simulink model "System_Design_Quadrocopter"  (Simulink 7.5)
settings: Solver=ode45  StartTime=0.0  StopTime=30  RelTol=1e-3
values from neighbouring files (symbols this model uses):
  phi0 = 0.15    [Quadrocopter_control_Driver.m]    (also in calc_stability.m = 0)
  r_phi0 = 0    [Quadrocopter_control_Driver.m]    (also in calc_stability.m)
  r_psi0 = 0    [Quadrocopter_control_Driver.m]    (also in calc_stability.m)
  r_theta0 = 0    [Quadrocopter_control_Driver.m]    (also in calc_stability.m)
  theta0 = 0.15    [Quadrocopter_control_Driver.m]    (also in calc_stability.m = 0)
  Ts = 0.01    [Reglerauslegung.m]    (also in Test_Reglerauslegung.m)
undefined symbols (not defined in the file or in its folder): bodyCtrl_phiCtrl_KD, bodyCtrl_phiCtrl_KI, bodyCtrl_phiCtrl_KP, bodyCtrl_rphiCtrl_KD, bodyCtrl_rphiCtrl_KI, bodyCtrl_rphiCtrl_KP, bodyCtrl_rpsiCtrl_KD, bodyCtrl_rpsiCtrl_KI, bodyCtrl_rpsiCtrl_KP, bodyCtrl_rthetaCtrl_KD, bodyCtrl_rthetaCtrl_KI, bodyCtrl_rthetaCtrl_KP, bodyCtrl_thetaCtrl_KD, bodyCtrl_thetaCtrl_KI, bodyCtrl_thetaCtrl_KP, boom, f1, f2, f3, f4, f5, g, I_x, I_y, I_z, m, positionCtrl_rpsiCtrl_KD, positionCtrl_rpsiCtrl_KI, positionCtrl_rpsiCtrl_KP, sigbuilder_block, speed, thrust, Ts_Opt
libraries: simulink x39, dspobslib x4, Copter_Library x3, Control_lib x1, sdolib x1
(part 2 of 4)

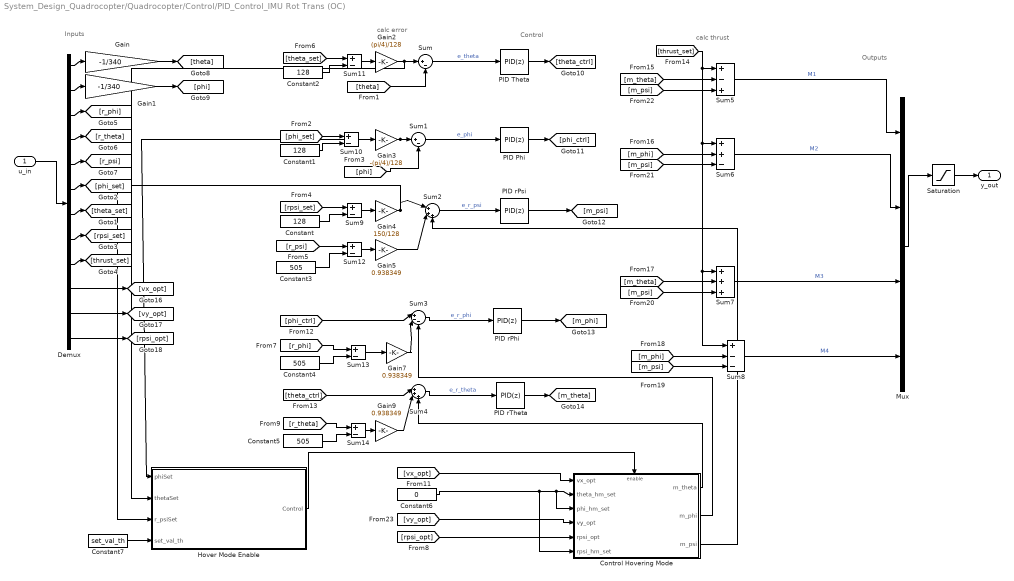
== system System_Design_Quadrocopter/Quadrocopter/Control/PID_Control_IMU Rot Trans (OC) ==
  note: calc thrust
  note: Control
  note: Outputs
  note: calc error
  note: Inputs
  u_in : Inport  OutDataType=fixdt(1, 16)  OutScaling=2^0
  Constant : Constant  Value=128  OutDataType=fixdt(1, 16)  OutScaling=2^0
  Constant1 : Constant  Value=128  OutDataType=fixdt(1, 16)  OutScaling=2^0
  Constant2 : Constant  Value=128  OutDataType=fixdt(1, 16)  OutScaling=2^0
  Constant3 : Constant  Value=505  OutDataType=fixdt(1, 16)  OutScaling=2^0
  Constant4 : Constant  Value=505  OutDataType=fixdt(1, 16)  OutScaling=2^0
  Constant5 : Constant  Value=505  OutDataType=fixdt(1, 16)  OutScaling=2^0
  Constant6 : Constant  Value=0  OutDataType=fixdt(1, 16)  OutScaling=2^0
  Constant7 : Constant  Value=set_val_th  OutDataType=fixdt(1, 16)  OutScaling=2^0
  Control Hovering Mode : Subsystem
  Demux : Demux  Outputs=12
  Gain : Gain  Gain=-1/340  ParameterDataType=fixdt(1, 16)  ParameterScaling=2^0  OutDataType=fixdt(1, 16)  OutScaling=2^0
  Gain1 : Gain  Gain=-1/340  ParameterDataType=fixdt(1, 16)  ParameterScaling=2^0  OutDataType=fixdt(1, 16)  OutScaling=2^0
  Gain2 : Gain  Gain=(pi/4)/128  ParameterDataType=fixdt(1, 16)  ParameterScaling=2^0  OutDataType=fixdt(1, 16)  OutScaling=2^0
  Gain3 : Gain  Gain=-(pi/4)/128  ParameterDataType=fixdt(1, 16)  ParameterScaling=2^0  OutDataType=fixdt(1, 16)  OutScaling=2^0
  Gain4 : Gain  Gain=150/128  ParameterDataType=fixdt(1, 16)  ParameterScaling=2^0  OutDataType=fixdt(1, 16)  OutScaling=2^0
  Gain5 : Gain  Gain=0.938349  ParameterDataType=fixdt(1, 16)  ParameterScaling=2^0  OutDataType=fixdt(1, 16)  OutScaling=2^0
  Gain7 : Gain  Gain=0.938349  ParameterDataType=fixdt(1, 16)  ParameterScaling=2^0  OutDataType=fixdt(1, 16)  OutScaling=2^0
  Gain9 : Gain  Gain=0.938349  ParameterDataType=fixdt(1, 16)  ParameterScaling=2^0  OutDataType=fixdt(1, 16)  OutScaling=2^0
  Hover Mode Enable : Stateflow chart  TreatAsAtomicUnit=on
  Mux : Mux
  PID Phi : simulink/Continuous/PID Controller  DialogController=pidpack.PIDConfig.pidDDGCreate  DialogControllerArgs=DataTag9  SystemSampleTime=-1  Controller=PID  TimeDomain=Discrete-time  SampleTime=Ts  IntegratorMethod=Forward Euler  FilterMethod=Forward Euler  Form=Ideal  P=150  I=0.5  D=0  N=0  InitialConditionSource=internal  InitialConditionForIntegrator=0  InitialConditionForFilter=0  ExternalReset=none  ZeroCross=off  LimitOutput=off  UpperSaturationLimit=inf  LowerSaturationLimit=-inf  LinearizeAsGain=off  AntiWindupMode=none  Kb=1  TrackingMode=off  Kt=1  PParamMin=[]  PParamMax=[]  IParamMin=[]  IParamMax=[]  DParamMin=[]  DParamMax=[]  NParamMin=[]  NParamMax=[]  KbParamMin=[]  KbParamMax=[]  KtParamMin=[]  KtParamMax=[]  POutMin=[]  POutMax=[]  IOutMin=[]  IOutMax=[]  DOutMin=[]  DOutMax=[]  NOutMin=[]  NOutMax=[]  KbOutMin=[]  KbOutMax=[]  KtOutMin=[]  KtOutMax=[]  IntegratorOutMin=[]  IntegratorOutMax=[]  FilterOutMin=[]  FilterOutMax=[]  SumOutMin=[]  SumOutMax=[]  SumI1OutMin=[]  SumI1OutMax=[]  SumI2OutMin=[]  SumI2OutMax=[]  SumI3OutMin=[]  SumI3OutMax=[]  SumDOutMin=[]  SumDOutMax=[]  SaturationOutMin=[]  SaturationOutMax=[]  IntegratorContinuousStateAttributes=''  IntegratorStateMustResolveToSignalObject=off  IntegratorRTWStateStorageClass=Auto  FilterContinuousStateAttributes=''  FilterStateMustResolveToSignalObject=off  FilterRTWStateStorageClass=Auto
  PID Theta : simulink/Continuous/PID Controller  DialogController=pidpack.PIDConfig.pidDDGCreate  DialogControllerArgs=DataTag10  SystemSampleTime=-1  Controller=PID  TimeDomain=Discrete-time  SampleTime=Ts  IntegratorMethod=Forward Euler  FilterMethod=Forward Euler  Form=Ideal  P=150  I=0.5  D=0  N=0  InitialConditionSource=internal  InitialConditionForIntegrator=0  InitialConditionForFilter=0  ExternalReset=none  ZeroCross=off  LimitOutput=off  UpperSaturationLimit=inf  LowerSaturationLimit=-inf  LinearizeAsGain=off  AntiWindupMode=none  Kb=1  TrackingMode=off  Kt=1  PParamMin=[]  PParamMax=[]  IParamMin=[]  IParamMax=[]  DParamMin=[]  DParamMax=[]  NParamMin=[]  NParamMax=[]  KbParamMin=[]  KbParamMax=[]  KtParamMin=[]  KtParamMax=[]  POutMin=[]  POutMax=[]  IOutMin=[]  IOutMax=[]  DOutMin=[]  DOutMax=[]  NOutMin=[]  NOutMax=[]  KbOutMin=[]  KbOutMax=[]  KtOutMin=[]  KtOutMax=[]  IntegratorOutMin=[]  IntegratorOutMax=[]  FilterOutMin=[]  FilterOutMax=[]  SumOutMin=[]  SumOutMax=[]  SumI1OutMin=[]  SumI1OutMax=[]  SumI2OutMin=[]  SumI2OutMax=[]  SumI3OutMin=[]  SumI3OutMax=[]  SumDOutMin=[]  SumDOutMax=[]  SaturationOutMin=[]  SaturationOutMax=[]  IntegratorContinuousStateAttributes=''  IntegratorStateMustResolveToSignalObject=off  IntegratorRTWStateStorageClass=Auto  FilterContinuousStateAttributes=''  FilterStateMustResolveToSignalObject=off  FilterRTWStateStorageClass=Auto
  PID rPhi : simulink/Continuous/PID Controller  DialogController=pidpack.PIDConfig.pidDDGCreate  DialogControllerArgs=DataTag11  SystemSampleTime=-1  Controller=PID  TimeDomain=Discrete-time  SampleTime=Ts  IntegratorMethod=Forward Euler  FilterMethod=Forward Euler  Form=Ideal  P=60  I=0.5  D=0  N=0  InitialConditionSource=internal  InitialConditionForIntegrator=0  InitialConditionForFilter=0  ExternalReset=none  ZeroCross=off  LimitOutput=off  UpperSaturationLimit=inf  LowerSaturationLimit=-inf  LinearizeAsGain=off  AntiWindupMode=none  Kb=1  TrackingMode=off  Kt=1  PParamMin=[]  PParamMax=[]  IParamMin=[]  IParamMax=[]  DParamMin=[]  DParamMax=[]  NParamMin=[]  NParamMax=[]  KbParamMin=[]  KbParamMax=[]  KtParamMin=[]  KtParamMax=[]  POutMin=[]  POutMax=[]  IOutMin=[]  IOutMax=[]  DOutMin=[]  DOutMax=[]  NOutMin=[]  NOutMax=[]  KbOutMin=[]  KbOutMax=[]  KtOutMin=[]  KtOutMax=[]  IntegratorOutMin=[]  IntegratorOutMax=[]  FilterOutMin=[]  FilterOutMax=[]  SumOutMin=[]  SumOutMax=[]  SumI1OutMin=[]  SumI1OutMax=[]  SumI2OutMin=[]  SumI2OutMax=[]  SumI3OutMin=[]  SumI3OutMax=[]  SumDOutMin=[]  SumDOutMax=[]  SaturationOutMin=[]  SaturationOutMax=[]  IntegratorContinuousStateAttributes=''  IntegratorStateMustResolveToSignalObject=off  IntegratorRTWStateStorageClass=Auto  FilterContinuousStateAttributes=''  FilterStateMustResolveToSignalObject=off  FilterRTWStateStorageClass=Auto
  PID rPsi : simulink/Continuous/PID Controller  DialogController=pidpack.PIDConfig.pidDDGCreate  DialogControllerArgs=DataTag12  SystemSampleTime=-1  Controller=PID  TimeDomain=Discrete-time  SampleTime=Ts  IntegratorMethod=Forward Euler  FilterMethod=Forward Euler  Form=Ideal  P=60  I=0  D=0  N=0  InitialConditionSource=internal  InitialConditionForIntegrator=0  InitialConditionForFilter=0  ExternalReset=none  ZeroCross=off  LimitOutput=off  UpperSaturationLimit=inf  LowerSaturationLimit=-inf  LinearizeAsGain=off  AntiWindupMode=none  Kb=1  TrackingMode=off  Kt=1  PParamMin=[]  PParamMax=[]  IParamMin=[]  IParamMax=[]  DParamMin=[]  DParamMax=[]  NParamMin=[]  NParamMax=[]  KbParamMin=[]  KbParamMax=[]  KtParamMin=[]  KtParamMax=[]  POutMin=[]  POutMax=[]  IOutMin=[]  IOutMax=[]  DOutMin=[]  DOutMax=[]  NOutMin=[]  NOutMax=[]  KbOutMin=[]  KbOutMax=[]  KtOutMin=[]  KtOutMax=[]  IntegratorOutMin=[]  IntegratorOutMax=[]  FilterOutMin=[]  FilterOutMax=[]  SumOutMin=[]  SumOutMax=[]  SumI1OutMin=[]  SumI1OutMax=[]  SumI2OutMin=[]  SumI2OutMax=[]  SumI3OutMin=[]  SumI3OutMax=[]  SumDOutMin=[]  SumDOutMax=[]  SaturationOutMin=[]  SaturationOutMax=[]  IntegratorContinuousStateAttributes=''  IntegratorStateMustResolveToSignalObject=off  IntegratorRTWStateStorageClass=Auto  FilterContinuousStateAttributes=''  FilterStateMustResolveToSignalObject=off  FilterRTWStateStorageClass=Auto
  PID rTheta : simulink/Continuous/PID Controller  DialogController=pidpack.PIDConfig.pidDDGCreate  DialogControllerArgs=DataTag13  SystemSampleTime=-1  Controller=PID  TimeDomain=Discrete-time  SampleTime=Ts  IntegratorMethod=Forward Euler  FilterMethod=Forward Euler  Form=Ideal  P=60  I=0.5  D=0  N=0  InitialConditionSource=internal  InitialConditionForIntegrator=0  InitialConditionForFilter=0  ExternalReset=none  ZeroCross=off  LimitOutput=off  UpperSaturationLimit=inf  LowerSaturationLimit=-inf  LinearizeAsGain=off  AntiWindupMode=none  Kb=1  TrackingMode=off  Kt=1  PParamMin=[]  PParamMax=[]  IParamMin=[]  IParamMax=[]  DParamMin=[]  DParamMax=[]  NParamMin=[]  NParamMax=[]  KbParamMin=[]  KbParamMax=[]  KtParamMin=[]  KtParamMax=[]  POutMin=[]  POutMax=[]  IOutMin=[]  IOutMax=[]  DOutMin=[]  DOutMax=[]  NOutMin=[]  NOutMax=[]  KbOutMin=[]  KbOutMax=[]  KtOutMin=[]  KtOutMax=[]  IntegratorOutMin=[]  IntegratorOutMax=[]  FilterOutMin=[]  FilterOutMax=[]  SumOutMin=[]  SumOutMax=[]  SumI1OutMin=[]  SumI1OutMax=[]  SumI2OutMin=[]  SumI2OutMax=[]  SumI3OutMin=[]  SumI3OutMax=[]  SumDOutMin=[]  SumDOutMax=[]  SaturationOutMin=[]  SaturationOutMax=[]  IntegratorContinuousStateAttributes=''  IntegratorStateMustResolveToSignalObject=off  IntegratorRTWStateStorageClass=Auto  FilterContinuousStateAttributes=''  FilterStateMustResolveToSignalObject=off  FilterRTWStateStorageClass=Auto
  Saturation : Saturate  UpperLimit=255  LowerLimit=0  OutDataType=fixdt(1, 16)  OutScaling=2^0
  Sum : Sum  Inputs=|+-  OutDataType=fixdt(1, 16)  OutScaling=2^0
  Sum1 : Sum  Inputs=|+-  OutDataType=fixdt(1, 16)  OutScaling=2^0
  Sum{9..14} (6 alike) : Sum  Inputs=+-  OutDataType=fixdt(1, 16)  OutScaling=2^0
  Sum2 : Sum  Inputs=|+++  OutDataType=fixdt(1, 16)  OutScaling=2^0
  Sum3 : Sum  Inputs=|+--  OutDataType=fixdt(1, 16)  OutScaling=2^0
  Sum4 : Sum  Inputs=|+++  OutDataType=fixdt(1, 16)  OutScaling=2^0
  Sum5 : Sum  Inputs=+-+  OutDataType=fixdt(1, 16)  OutScaling=2^0
  Sum6 : Sum  Inputs=++-  OutDataType=fixdt(1, 16)  OutScaling=2^0
  Sum7 : Sum  Inputs=+++  OutDataType=fixdt(1, 16)  OutScaling=2^0
  Sum8 : Sum  Inputs=+--  OutDataType=fixdt(1, 16)  OutScaling=2^0
  y_out : Outport  OutDataType=fixdt(1, 16)  OutScaling=2^0
  wires:
  Gain4/1 -> Hover Mode Enable/3(r_psiSet), Sum2/1
  Sum9/1 -> Gain4/1
  [phi_ctrl] -> Sum3/1
  Sum14/1 -> Gain9/1
  Gain9/1 -> Sum4/2
  [theta_ctrl] -> Sum4/1
  Sum13/1 -> Gain7/1
  Gain7/1 -> Sum3/2
  Gain3/1 -> Sum1/1, Hover Mode Enable/1(phiSet)
  Gain2/1 -> Sum/1, Hover Mode Enable/2(thetaSet)
  Sum11/1 -> Gain2/1
  Sum10/1 -> Gain3/1
  [r_theta] -> Sum14/1
  Constant5/1 -> Sum14/2
  [r_phi] -> Sum13/1
  Constant4/1 -> Sum13/2
  Constant2/1 -> Sum11/2
  [theta_set] -> Sum11/1
  Constant1/1 -> Sum10/2
  [phi_set] -> Sum10/1
  Constant/1 -> Sum9/2
  [rpsi_set] -> Sum9/1
  Saturation/1 -> y_out/1
  Mux/1 -> Saturation/1
  [m_psi] -> Sum8/3
  [m_phi] -> Sum8/2
  [m_psi] -> Sum7/3
  [m_theta] -> Sum7/2
  [m_psi] -> Sum6/3
  [m_phi] -> Sum6/2
  [m_psi] -> Sum5/3
  [m_theta] -> Sum5/2
  [thrust_set] -> Sum8/1, Sum7/1, Sum6/1, Sum5/1
  PID rTheta/1 -> [m_theta]
  PID rPhi/1 -> [m_phi]
  PID Theta/1 -> [theta_ctrl]
  PID Phi/1 -> [phi_ctrl]
  Sum6/1 -> Mux/2  "M2"
  Sum7/1 -> Mux/3  "M3"
  Sum8/1 -> Mux/4  "M4"
  Sum5/1 -> Mux/1  "M1"
  Sum4/1 -> PID rTheta/1  "e_r_theta"
  Sum3/1 -> PID rPhi/1  "e_r_phi"
  Sum2/1 -> PID rPsi/1  "e_r_psi"
  Sum1/1 -> PID Phi/1  "e_phi"
  [phi] -> Sum1/2
  Sum/1 -> PID Theta/1  "e_theta"
  [theta] -> Sum/2
  Gain1/1 -> [phi]
  Gain/1 -> [theta]
  Demux/9 -> [thrust_set]
  Demux/8 -> [rpsi_set]
  Demux/7 -> [theta_set]
  Demux/6 -> [phi_set]
  Demux/5 -> [r_psi]
  Demux/4 -> [r_theta]
  Demux/3 -> [r_phi]
  Demux/1 -> Gain/1
  Demux/2 -> Gain1/1
  u_in/1 -> Demux/1
  Demux/10 -> [vx_opt]
  Demux/11 -> [vy_opt]
  Demux/12 -> [rpsi_opt]
  [vy_opt] -> Control Hovering Mode/4(vy_opt)
  [vx_opt] -> Control Hovering Mode/1(vx_opt)
  [rpsi_opt] -> Control Hovering Mode/5(rpsi_opt)
  Control Hovering Mode/1(m_theta) -> Sum4/3
  Control Hovering Mode/2(m_phi) -> Sum3/3
  Constant7/1 -> Hover Mode Enable/4(set_val_th)
  Gain5/1 -> Sum2/2
  Sum12/1 -> Gain5/1
  Constant3/1 -> Sum12/2
  [r_psi] -> Sum12/1
  Constant6/1 -> Control Hovering Mode/2(theta_hm_set), Control Hovering Mode/3(phi_hm_set), Control Hovering Mode/6(rpsi_hm_set)
  PID rPsi/1 -> [m_psi]
  Hover Mode Enable/1(Control) -> Control Hovering Mode/Enable
  Control Hovering Mode/3(m_psi) -> Sum2/3

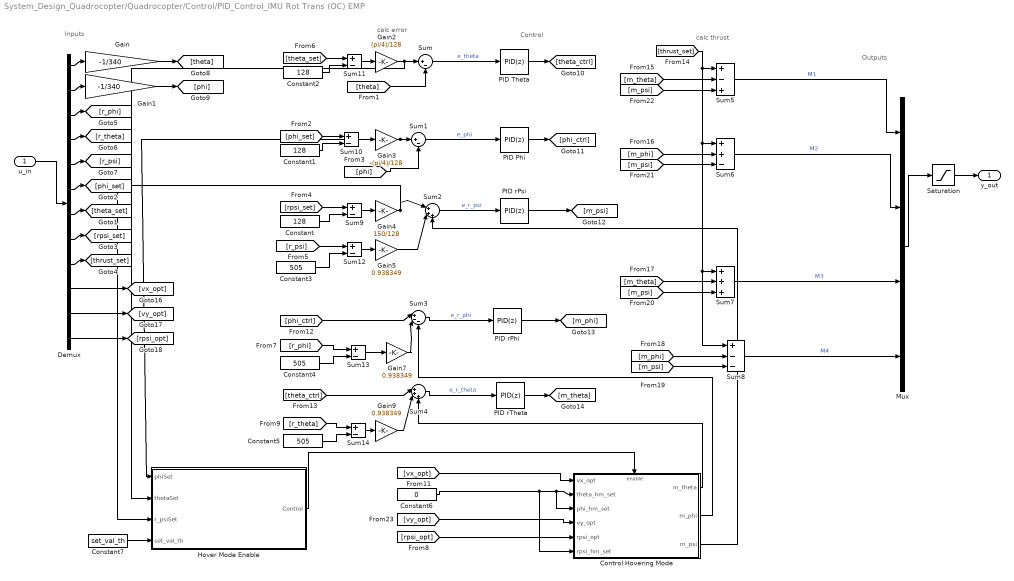
== system System_Design_Quadrocopter/Quadrocopter/Control/PID_Control_IMU Rot Trans (OC) EMP ==
  note: calc thrust
  note: Control
  note: Outputs
  note: calc error
  note: Inputs
  u_in : Inport  OutDataType=fixdt(1, 16)  OutScaling=2^0
  Constant : Constant  Value=128  OutDataType=fixdt(1, 16)  OutScaling=2^0
  Constant1 : Constant  Value=128  OutDataType=fixdt(1, 16)  OutScaling=2^0
  Constant2 : Constant  Value=128  OutDataType=fixdt(1, 16)  OutScaling=2^0
  Constant3 : Constant  Value=505  OutDataType=fixdt(1, 16)  OutScaling=2^0
  Constant4 : Constant  Value=505  OutDataType=fixdt(1, 16)  OutScaling=2^0
  Constant5 : Constant  Value=505  OutDataType=fixdt(1, 16)  OutScaling=2^0
  Constant6 : Constant  Value=0  OutDataType=fixdt(1, 16)  OutScaling=2^0
  Constant7 : Constant  Value=set_val_th  OutDataType=fixdt(1, 16)  OutScaling=2^0
  Control Hovering Mode : Subsystem
  Demux : Demux  Outputs=12
  Gain : Gain  Gain=-1/340  ParameterDataType=fixdt(1, 16)  ParameterScaling=2^0  OutDataType=fixdt(1, 16)  OutScaling=2^0
  Gain1 : Gain  Gain=-1/340  ParameterDataType=fixdt(1, 16)  ParameterScaling=2^0  OutDataType=fixdt(1, 16)  OutScaling=2^0
  Gain2 : Gain  Gain=(pi/4)/128  ParameterDataType=fixdt(1, 16)  ParameterScaling=2^0  OutDataType=fixdt(1, 16)  OutScaling=2^0
  Gain3 : Gain  Gain=-(pi/4)/128  ParameterDataType=fixdt(1, 16)  ParameterScaling=2^0  OutDataType=fixdt(1, 16)  OutScaling=2^0
  Gain4 : Gain  Gain=150/128  ParameterDataType=fixdt(1, 16)  ParameterScaling=2^0  OutDataType=fixdt(1, 16)  OutScaling=2^0
  Gain5 : Gain  Gain=0.938349  ParameterDataType=fixdt(1, 16)  ParameterScaling=2^0  OutDataType=fixdt(1, 16)  OutScaling=2^0
  Gain7 : Gain  Gain=0.938349  ParameterDataType=fixdt(1, 16)  ParameterScaling=2^0  OutDataType=fixdt(1, 16)  OutScaling=2^0
  Gain9 : Gain  Gain=0.938349  ParameterDataType=fixdt(1, 16)  ParameterScaling=2^0  OutDataType=fixdt(1, 16)  OutScaling=2^0
  Hover Mode Enable : Stateflow chart  TreatAsAtomicUnit=on
  Mux : Mux
  PID Phi : simulink/Continuous/PID Controller  DialogController=pidpack.PIDConfig.pidDDGCreate  DialogControllerArgs=DataTag17  SystemSampleTime=-1  Controller=PID  TimeDomain=Discrete-time  SampleTime=Ts  IntegratorMethod=Forward Euler  FilterMethod=Forward Euler  Form=Ideal  P=bodyCtrl_phiCtrl_KP  I=bodyCtrl_phiCtrl_KI  D=bodyCtrl_phiCtrl_KD  N=0  InitialConditionSource=internal  InitialConditionForIntegrator=0  InitialConditionForFilter=0  ExternalReset=none  ZeroCross=off  LimitOutput=off  UpperSaturationLimit=inf  LowerSaturationLimit=-inf  LinearizeAsGain=off  AntiWindupMode=none  Kb=1  TrackingMode=off  Kt=1  PParamMin=[]  PParamMax=[]  IParamMin=[]  IParamMax=[]  DParamMin=[]  DParamMax=[]  NParamMin=[]  NParamMax=[]  KbParamMin=[]  KbParamMax=[]  KtParamMin=[]  KtParamMax=[]  POutMin=[]  POutMax=[]  IOutMin=[]  IOutMax=[]  DOutMin=[]  DOutMax=[]  NOutMin=[]  NOutMax=[]  KbOutMin=[]  KbOutMax=[]  KtOutMin=[]  KtOutMax=[]  IntegratorOutMin=[]  IntegratorOutMax=[]  FilterOutMin=[]  FilterOutMax=[]  SumOutMin=[]  SumOutMax=[]  SumI1OutMin=[]  SumI1OutMax=[]  SumI2OutMin=[]  SumI2OutMax=[]  SumI3OutMin=[]  SumI3OutMax=[]  SumDOutMin=[]  SumDOutMax=[]  SaturationOutMin=[]  SaturationOutMax=[]  IntegratorContinuousStateAttributes=''  IntegratorStateMustResolveToSignalObject=off  IntegratorRTWStateStorageClass=Auto  FilterContinuousStateAttributes=''  FilterStateMustResolveToSignalObject=off  FilterRTWStateStorageClass=Auto
  PID Theta : simulink/Continuous/PID Controller  DialogController=pidpack.PIDConfig.pidDDGCreate  DialogControllerArgs=DataTag18  SystemSampleTime=-1  Controller=PID  TimeDomain=Discrete-time  SampleTime=Ts  IntegratorMethod=Forward Euler  FilterMethod=Forward Euler  Form=Ideal  P=bodyCtrl_thetaCtrl_KP  I=bodyCtrl_thetaCtrl_KI  D=bodyCtrl_thetaCtrl_KD  N=0  InitialConditionSource=internal  InitialConditionForIntegrator=0  InitialConditionForFilter=0  ExternalReset=none  ZeroCross=off  LimitOutput=off  UpperSaturationLimit=inf  LowerSaturationLimit=-inf  LinearizeAsGain=off  AntiWindupMode=none  Kb=1  TrackingMode=off  Kt=1  PParamMin=[]  PParamMax=[]  IParamMin=[]  IParamMax=[]  DParamMin=[]  DParamMax=[]  NParamMin=[]  NParamMax=[]  KbParamMin=[]  KbParamMax=[]  KtParamMin=[]  KtParamMax=[]  POutMin=[]  POutMax=[]  IOutMin=[]  IOutMax=[]  DOutMin=[]  DOutMax=[]  NOutMin=[]  NOutMax=[]  KbOutMin=[]  KbOutMax=[]  KtOutMin=[]  KtOutMax=[]  IntegratorOutMin=[]  IntegratorOutMax=[]  FilterOutMin=[]  FilterOutMax=[]  SumOutMin=[]  SumOutMax=[]  SumI1OutMin=[]  SumI1OutMax=[]  SumI2OutMin=[]  SumI2OutMax=[]  SumI3OutMin=[]  SumI3OutMax=[]  SumDOutMin=[]  SumDOutMax=[]  SaturationOutMin=[]  SaturationOutMax=[]  IntegratorContinuousStateAttributes=''  IntegratorStateMustResolveToSignalObject=off  IntegratorRTWStateStorageClass=Auto  FilterContinuousStateAttributes=''  FilterStateMustResolveToSignalObject=off  FilterRTWStateStorageClass=Auto
  PID rPhi : simulink/Continuous/PID Controller  DialogController=pidpack.PIDConfig.pidDDGCreate  DialogControllerArgs=DataTag19  SystemSampleTime=-1  Controller=PID  TimeDomain=Discrete-time  SampleTime=Ts  IntegratorMethod=Forward Euler  FilterMethod=Forward Euler  Form=Ideal  P=bodyCtrl_rphiCtrl_KP  I=bodyCtrl_rphiCtrl_KI  D=bodyCtrl_rphiCtrl_KD  N=0  InitialConditionSource=internal  InitialConditionForIntegrator=0  InitialConditionForFilter=0  ExternalReset=none  ZeroCross=off  LimitOutput=off  UpperSaturationLimit=inf  LowerSaturationLimit=-inf  LinearizeAsGain=off  AntiWindupMode=none  Kb=1  TrackingMode=off  Kt=1  PParamMin=[]  PParamMax=[]  IParamMin=[]  IParamMax=[]  DParamMin=[]  DParamMax=[]  NParamMin=[]  NParamMax=[]  KbParamMin=[]  KbParamMax=[]  KtParamMin=[]  KtParamMax=[]  POutMin=[]  POutMax=[]  IOutMin=[]  IOutMax=[]  DOutMin=[]  DOutMax=[]  NOutMin=[]  NOutMax=[]  KbOutMin=[]  KbOutMax=[]  KtOutMin=[]  KtOutMax=[]  IntegratorOutMin=[]  IntegratorOutMax=[]  FilterOutMin=[]  FilterOutMax=[]  SumOutMin=[]  SumOutMax=[]  SumI1OutMin=[]  SumI1OutMax=[]  SumI2OutMin=[]  SumI2OutMax=[]  SumI3OutMin=[]  SumI3OutMax=[]  SumDOutMin=[]  SumDOutMax=[]  SaturationOutMin=[]  SaturationOutMax=[]  IntegratorContinuousStateAttributes=''  IntegratorStateMustResolveToSignalObject=off  IntegratorRTWStateStorageClass=Auto  FilterContinuousStateAttributes=''  FilterStateMustResolveToSignalObject=off  FilterRTWStateStorageClass=Auto
  PID rPsi : simulink/Continuous/PID Controller  DialogController=pidpack.PIDConfig.pidDDGCreate  DialogControllerArgs=DataTag20  SystemSampleTime=-1  Controller=PID  TimeDomain=Discrete-time  SampleTime=Ts  IntegratorMethod=Forward Euler  FilterMethod=Forward Euler  Form=Ideal  P=bodyCtrl_rpsiCtrl_KP  I=bodyCtrl_rpsiCtrl_KI  D=bodyCtrl_rpsiCtrl_KD  N=0  InitialConditionSource=internal  InitialConditionForIntegrator=0  InitialConditionForFilter=0  ExternalReset=none  ZeroCross=off  LimitOutput=off  UpperSaturationLimit=inf  LowerSaturationLimit=-inf  LinearizeAsGain=off  AntiWindupMode=none  Kb=1  TrackingMode=off  Kt=1  PParamMin=[]  PParamMax=[]  IParamMin=[]  IParamMax=[]  DParamMin=[]  DParamMax=[]  NParamMin=[]  NParamMax=[]  KbParamMin=[]  KbParamMax=[]  KtParamMin=[]  KtParamMax=[]  POutMin=[]  POutMax=[]  IOutMin=[]  IOutMax=[]  DOutMin=[]  DOutMax=[]  NOutMin=[]  NOutMax=[]  KbOutMin=[]  KbOutMax=[]  KtOutMin=[]  KtOutMax=[]  IntegratorOutMin=[]  IntegratorOutMax=[]  FilterOutMin=[]  FilterOutMax=[]  SumOutMin=[]  SumOutMax=[]  SumI1OutMin=[]  SumI1OutMax=[]  SumI2OutMin=[]  SumI2OutMax=[]  SumI3OutMin=[]  SumI3OutMax=[]  SumDOutMin=[]  SumDOutMax=[]  SaturationOutMin=[]  SaturationOutMax=[]  IntegratorContinuousStateAttributes=''  IntegratorStateMustResolveToSignalObject=off  IntegratorRTWStateStorageClass=Auto  FilterContinuousStateAttributes=''  FilterStateMustResolveToSignalObject=off  FilterRTWStateStorageClass=Auto
  PID rTheta : simulink/Continuous/PID Controller  DialogController=pidpack.PIDConfig.pidDDGCreate  DialogControllerArgs=DataTag21  SystemSampleTime=-1  Controller=PID  TimeDomain=Discrete-time  SampleTime=Ts  IntegratorMethod=Forward Euler  FilterMethod=Forward Euler  Form=Ideal  P=bodyCtrl_rthetaCtrl_KP  I=bodyCtrl_rthetaCtrl_KI  D=bodyCtrl_rthetaCtrl_KD  N=0  InitialConditionSource=internal  InitialConditionForIntegrator=0  InitialConditionForFilter=0  ExternalReset=none  ZeroCross=off  LimitOutput=off  UpperSaturationLimit=inf  LowerSaturationLimit=-inf  LinearizeAsGain=off  AntiWindupMode=none  Kb=1  TrackingMode=off  Kt=1  PParamMin=[]  PParamMax=[]  IParamMin=[]  IParamMax=[]  DParamMin=[]  DParamMax=[]  NParamMin=[]  NParamMax=[]  KbParamMin=[]  KbParamMax=[]  KtParamMin=[]  KtParamMax=[]  POutMin=[]  POutMax=[]  IOutMin=[]  IOutMax=[]  DOutMin=[]  DOutMax=[]  NOutMin=[]  NOutMax=[]  KbOutMin=[]  KbOutMax=[]  KtOutMin=[]  KtOutMax=[]  IntegratorOutMin=[]  IntegratorOutMax=[]  FilterOutMin=[]  FilterOutMax=[]  SumOutMin=[]  SumOutMax=[]  SumI1OutMin=[]  SumI1OutMax=[]  SumI2OutMin=[]  SumI2OutMax=[]  SumI3OutMin=[]  SumI3OutMax=[]  SumDOutMin=[]  SumDOutMax=[]  SaturationOutMin=[]  SaturationOutMax=[]  IntegratorContinuousStateAttributes=''  IntegratorStateMustResolveToSignalObject=off  IntegratorRTWStateStorageClass=Auto  FilterContinuousStateAttributes=''  FilterStateMustResolveToSignalObject=off  FilterRTWStateStorageClass=Auto
  Saturation : Saturate  UpperLimit=255  LowerLimit=0  OutDataType=fixdt(1, 16)  OutScaling=2^0
  Sum : Sum  Inputs=|+-  OutDataType=fixdt(1, 16)  OutScaling=2^0
  Sum1 : Sum  Inputs=|+-  OutDataType=fixdt(1, 16)  OutScaling=2^0
  Sum{9..14} (6 alike) : Sum  Inputs=+-  OutDataType=fixdt(1, 16)  OutScaling=2^0
  Sum2 : Sum  Inputs=|+++  OutDataType=fixdt(1, 16)  OutScaling=2^0
  Sum3 : Sum  Inputs=|+--  OutDataType=fixdt(1, 16)  OutScaling=2^0
  Sum4 : Sum  Inputs=|+++  OutDataType=fixdt(1, 16)  OutScaling=2^0
  Sum5 : Sum  Inputs=+-+  OutDataType=fixdt(1, 16)  OutScaling=2^0
  Sum6 : Sum  Inputs=++-  OutDataType=fixdt(1, 16)  OutScaling=2^0
  Sum7 : Sum  Inputs=+++  OutDataType=fixdt(1, 16)  OutScaling=2^0
  Sum8 : Sum  Inputs=+--  OutDataType=fixdt(1, 16)  OutScaling=2^0
  y_out : Outport  OutDataType=fixdt(1, 16)  OutScaling=2^0
  wires:
  Gain4/1 -> Hover Mode Enable/3(r_psiSet), Sum2/1
  Sum9/1 -> Gain4/1
  [phi_ctrl] -> Sum3/1
  Sum14/1 -> Gain9/1
  Gain9/1 -> Sum4/2
  [theta_ctrl] -> Sum4/1
  Sum13/1 -> Gain7/1
  Gain7/1 -> Sum3/2
  Gain3/1 -> Sum1/1, Hover Mode Enable/1(phiSet)
  Gain2/1 -> Sum/1, Hover Mode Enable/2(thetaSet)
  Sum11/1 -> Gain2/1
  Sum10/1 -> Gain3/1
  [r_theta] -> Sum14/1
  Constant5/1 -> Sum14/2
  [r_phi] -> Sum13/1
  Constant4/1 -> Sum13/2
  Constant2/1 -> Sum11/2
  [theta_set] -> Sum11/1
  Constant1/1 -> Sum10/2
  [phi_set] -> Sum10/1
  Constant/1 -> Sum9/2
  [rpsi_set] -> Sum9/1
  Saturation/1 -> y_out/1
  Mux/1 -> Saturation/1
  [m_psi] -> Sum8/3
  [m_phi] -> Sum8/2
  [m_psi] -> Sum7/3
  [m_theta] -> Sum7/2
  [m_psi] -> Sum6/3
  [m_phi] -> Sum6/2
  [m_psi] -> Sum5/3
  [m_theta] -> Sum5/2
  [thrust_set] -> Sum8/1, Sum7/1, Sum6/1, Sum5/1
  PID rTheta/1 -> [m_theta]
  PID rPhi/1 -> [m_phi]
  PID Theta/1 -> [theta_ctrl]
  PID Phi/1 -> [phi_ctrl]
  Sum6/1 -> Mux/2  "M2"
  Sum7/1 -> Mux/3  "M3"
  Sum8/1 -> Mux/4  "M4"
  Sum5/1 -> Mux/1  "M1"
  Sum4/1 -> PID rTheta/1  "e_r_theta"
  Sum3/1 -> PID rPhi/1  "e_r_phi"
  Sum2/1 -> PID rPsi/1  "e_r_psi"
  Sum1/1 -> PID Phi/1  "e_phi"
  [phi] -> Sum1/2
  Sum/1 -> PID Theta/1  "e_theta"
  [theta] -> Sum/2
  Gain1/1 -> [phi]
  Gain/1 -> [theta]
  Demux/9 -> [thrust_set]
  Demux/8 -> [rpsi_set]
  Demux/7 -> [theta_set]
  Demux/6 -> [phi_set]
  Demux/5 -> [r_psi]
  Demux/4 -> [r_theta]
  Demux/3 -> [r_phi]
  Demux/1 -> Gain/1
  Demux/2 -> Gain1/1
  u_in/1 -> Demux/1
  Demux/10 -> [vx_opt]
  Demux/11 -> [vy_opt]
  Demux/12 -> [rpsi_opt]
  [vy_opt] -> Control Hovering Mode/4(vy_opt)
  [vx_opt] -> Control Hovering Mode/1(vx_opt)
  [rpsi_opt] -> Control Hovering Mode/5(rpsi_opt)
  Control Hovering Mode/1(m_theta) -> Sum4/3
  Control Hovering Mode/2(m_phi) -> Sum3/3
  Constant7/1 -> Hover Mode Enable/4(set_val_th)
  Gain5/1 -> Sum2/2
  Sum12/1 -> Gain5/1
  Constant3/1 -> Sum12/2
  [r_psi] -> Sum12/1
  Constant6/1 -> Control Hovering Mode/2(theta_hm_set), Control Hovering Mode/3(phi_hm_set), Control Hovering Mode/6(rpsi_hm_set)
  PID rPsi/1 -> [m_psi]
  Hover Mode Enable/1(Control) -> Control Hovering Mode/Enable
  Control Hovering Mode/3(m_psi) -> Sum2/3

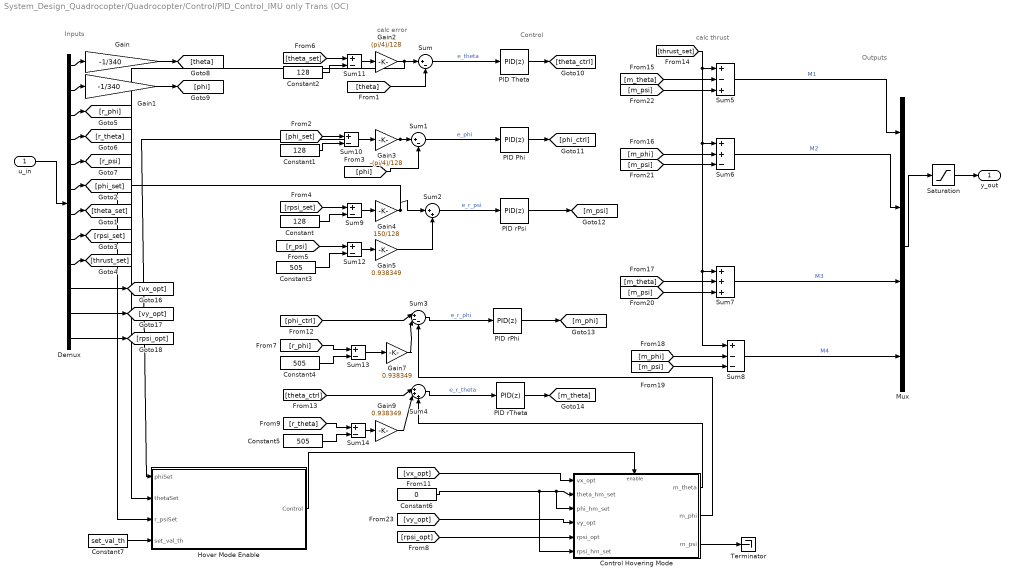
== system System_Design_Quadrocopter/Quadrocopter/Control/PID_Control_IMU only Trans (OC) ==
  note: calc thrust
  note: Control
  note: Outputs
  note: calc error
  note: Inputs
  u_in : Inport  OutDataType=fixdt(1, 16)  OutScaling=2^0
  Constant : Constant  Value=128  OutDataType=fixdt(1, 16)  OutScaling=2^0
  Constant1 : Constant  Value=128  OutDataType=fixdt(1, 16)  OutScaling=2^0
  Constant2 : Constant  Value=128  OutDataType=fixdt(1, 16)  OutScaling=2^0
  Constant3 : Constant  Value=505  OutDataType=fixdt(1, 16)  OutScaling=2^0
  Constant4 : Constant  Value=505  OutDataType=fixdt(1, 16)  OutScaling=2^0
  Constant5 : Constant  Value=505  OutDataType=fixdt(1, 16)  OutScaling=2^0
  Constant6 : Constant  Value=0  OutDataType=fixdt(1, 16)  OutScaling=2^0
  Constant7 : Constant  Value=set_val_th  OutDataType=fixdt(1, 16)  OutScaling=2^0
  Control Hovering Mode : Subsystem
  Demux : Demux  Outputs=12
  Gain : Gain  Gain=-1/340  ParameterDataType=fixdt(1, 16)  ParameterScaling=2^0  OutDataType=fixdt(1, 16)  OutScaling=2^0
  Gain1 : Gain  Gain=-1/340  ParameterDataType=fixdt(1, 16)  ParameterScaling=2^0  OutDataType=fixdt(1, 16)  OutScaling=2^0
  Gain2 : Gain  Gain=(pi/4)/128  ParameterDataType=fixdt(1, 16)  ParameterScaling=2^0  OutDataType=fixdt(1, 16)  OutScaling=2^0
  Gain3 : Gain  Gain=-(pi/4)/128  ParameterDataType=fixdt(1, 16)  ParameterScaling=2^0  OutDataType=fixdt(1, 16)  OutScaling=2^0
  Gain4 : Gain  Gain=150/128  ParameterDataType=fixdt(1, 16)  ParameterScaling=2^0  OutDataType=fixdt(1, 16)  OutScaling=2^0
  Gain5 : Gain  Gain=0.938349  ParameterDataType=fixdt(1, 16)  ParameterScaling=2^0  OutDataType=fixdt(1, 16)  OutScaling=2^0
  Gain7 : Gain  Gain=0.938349  ParameterDataType=fixdt(1, 16)  ParameterScaling=2^0  OutDataType=fixdt(1, 16)  OutScaling=2^0
  Gain9 : Gain  Gain=0.938349  ParameterDataType=fixdt(1, 16)  ParameterScaling=2^0  OutDataType=fixdt(1, 16)  OutScaling=2^0
  Hover Mode Enable : Stateflow chart  TreatAsAtomicUnit=on
  Mux : Mux
  PID Phi : simulink/Continuous/PID Controller  DialogController=pidpack.PIDConfig.pidDDGCreate  DialogControllerArgs=DataTag25  SystemSampleTime=-1  Controller=PID  TimeDomain=Discrete-time  SampleTime=Ts  IntegratorMethod=Forward Euler  FilterMethod=Forward Euler  Form=Ideal  P=150  I=0.5  D=0  N=0  InitialConditionSource=internal  InitialConditionForIntegrator=0  InitialConditionForFilter=0  ExternalReset=none  ZeroCross=off  LimitOutput=off  UpperSaturationLimit=inf  LowerSaturationLimit=-inf  LinearizeAsGain=off  AntiWindupMode=none  Kb=1  TrackingMode=off  Kt=1  PParamMin=[]  PParamMax=[]  IParamMin=[]  IParamMax=[]  DParamMin=[]  DParamMax=[]  NParamMin=[]  NParamMax=[]  KbParamMin=[]  KbParamMax=[]  KtParamMin=[]  KtParamMax=[]  POutMin=[]  POutMax=[]  IOutMin=[]  IOutMax=[]  DOutMin=[]  DOutMax=[]  NOutMin=[]  NOutMax=[]  KbOutMin=[]  KbOutMax=[]  KtOutMin=[]  KtOutMax=[]  IntegratorOutMin=[]  IntegratorOutMax=[]  FilterOutMin=[]  FilterOutMax=[]  SumOutMin=[]  SumOutMax=[]  SumI1OutMin=[]  SumI1OutMax=[]  SumI2OutMin=[]  SumI2OutMax=[]  SumI3OutMin=[]  SumI3OutMax=[]  SumDOutMin=[]  SumDOutMax=[]  SaturationOutMin=[]  SaturationOutMax=[]  IntegratorContinuousStateAttributes=''  IntegratorStateMustResolveToSignalObject=off  IntegratorRTWStateStorageClass=Auto  FilterContinuousStateAttributes=''  FilterStateMustResolveToSignalObject=off  FilterRTWStateStorageClass=Auto
  PID Theta : simulink/Continuous/PID Controller  DialogController=pidpack.PIDConfig.pidDDGCreate  DialogControllerArgs=DataTag26  SystemSampleTime=-1  Controller=PID  TimeDomain=Discrete-time  SampleTime=Ts  IntegratorMethod=Forward Euler  FilterMethod=Forward Euler  Form=Ideal  P=150  I=0.5  D=0  N=0  InitialConditionSource=internal  InitialConditionForIntegrator=0  InitialConditionForFilter=0  ExternalReset=none  ZeroCross=off  LimitOutput=off  UpperSaturationLimit=inf  LowerSaturationLimit=-inf  LinearizeAsGain=off  AntiWindupMode=none  Kb=1  TrackingMode=off  Kt=1  PParamMin=[]  PParamMax=[]  IParamMin=[]  IParamMax=[]  DParamMin=[]  DParamMax=[]  NParamMin=[]  NParamMax=[]  KbParamMin=[]  KbParamMax=[]  KtParamMin=[]  KtParamMax=[]  POutMin=[]  POutMax=[]  IOutMin=[]  IOutMax=[]  DOutMin=[]  DOutMax=[]  NOutMin=[]  NOutMax=[]  KbOutMin=[]  KbOutMax=[]  KtOutMin=[]  KtOutMax=[]  IntegratorOutMin=[]  IntegratorOutMax=[]  FilterOutMin=[]  FilterOutMax=[]  SumOutMin=[]  SumOutMax=[]  SumI1OutMin=[]  SumI1OutMax=[]  SumI2OutMin=[]  SumI2OutMax=[]  SumI3OutMin=[]  SumI3OutMax=[]  SumDOutMin=[]  SumDOutMax=[]  SaturationOutMin=[]  SaturationOutMax=[]  IntegratorContinuousStateAttributes=''  IntegratorStateMustResolveToSignalObject=off  IntegratorRTWStateStorageClass=Auto  FilterContinuousStateAttributes=''  FilterStateMustResolveToSignalObject=off  FilterRTWStateStorageClass=Auto
  PID rPhi : simulink/Continuous/PID Controller  DialogController=pidpack.PIDConfig.pidDDGCreate  DialogControllerArgs=DataTag27  SystemSampleTime=-1  Controller=PID  TimeDomain=Discrete-time  SampleTime=Ts  IntegratorMethod=Forward Euler  FilterMethod=Forward Euler  Form=Ideal  P=60  I=0.5  D=0  N=0  InitialConditionSource=internal  InitialConditionForIntegrator=0  InitialConditionForFilter=0  ExternalReset=none  ZeroCross=off  LimitOutput=off  UpperSaturationLimit=inf  LowerSaturationLimit=-inf  LinearizeAsGain=off  AntiWindupMode=none  Kb=1  TrackingMode=off  Kt=1  PParamMin=[]  PParamMax=[]  IParamMin=[]  IParamMax=[]  DParamMin=[]  DParamMax=[]  NParamMin=[]  NParamMax=[]  KbParamMin=[]  KbParamMax=[]  KtParamMin=[]  KtParamMax=[]  POutMin=[]  POutMax=[]  IOutMin=[]  IOutMax=[]  DOutMin=[]  DOutMax=[]  NOutMin=[]  NOutMax=[]  KbOutMin=[]  KbOutMax=[]  KtOutMin=[]  KtOutMax=[]  IntegratorOutMin=[]  IntegratorOutMax=[]  FilterOutMin=[]  FilterOutMax=[]  SumOutMin=[]  SumOutMax=[]  SumI1OutMin=[]  SumI1OutMax=[]  SumI2OutMin=[]  SumI2OutMax=[]  SumI3OutMin=[]  SumI3OutMax=[]  SumDOutMin=[]  SumDOutMax=[]  SaturationOutMin=[]  SaturationOutMax=[]  IntegratorContinuousStateAttributes=''  IntegratorStateMustResolveToSignalObject=off  IntegratorRTWStateStorageClass=Auto  FilterContinuousStateAttributes=''  FilterStateMustResolveToSignalObject=off  FilterRTWStateStorageClass=Auto
  PID rPsi : simulink/Continuous/PID Controller  DialogController=pidpack.PIDConfig.pidDDGCreate  DialogControllerArgs=DataTag28  SystemSampleTime=-1  Controller=PID  TimeDomain=Discrete-time  SampleTime=Ts  IntegratorMethod=Forward Euler  FilterMethod=Forward Euler  Form=Ideal  P=60  I=0  D=0  N=0  InitialConditionSource=internal  InitialConditionForIntegrator=0  InitialConditionForFilter=0  ExternalReset=none  ZeroCross=off  LimitOutput=off  UpperSaturationLimit=inf  LowerSaturationLimit=-inf  LinearizeAsGain=off  AntiWindupMode=none  Kb=1  TrackingMode=off  Kt=1  PParamMin=[]  PParamMax=[]  IParamMin=[]  IParamMax=[]  DParamMin=[]  DParamMax=[]  NParamMin=[]  NParamMax=[]  KbParamMin=[]  KbParamMax=[]  KtParamMin=[]  KtParamMax=[]  POutMin=[]  POutMax=[]  IOutMin=[]  IOutMax=[]  DOutMin=[]  DOutMax=[]  NOutMin=[]  NOutMax=[]  KbOutMin=[]  KbOutMax=[]  KtOutMin=[]  KtOutMax=[]  IntegratorOutMin=[]  IntegratorOutMax=[]  FilterOutMin=[]  FilterOutMax=[]  SumOutMin=[]  SumOutMax=[]  SumI1OutMin=[]  SumI1OutMax=[]  SumI2OutMin=[]  SumI2OutMax=[]  SumI3OutMin=[]  SumI3OutMax=[]  SumDOutMin=[]  SumDOutMax=[]  SaturationOutMin=[]  SaturationOutMax=[]  IntegratorContinuousStateAttributes=''  IntegratorStateMustResolveToSignalObject=off  IntegratorRTWStateStorageClass=Auto  FilterContinuousStateAttributes=''  FilterStateMustResolveToSignalObject=off  FilterRTWStateStorageClass=Auto
  PID rTheta : simulink/Continuous/PID Controller  DialogController=pidpack.PIDConfig.pidDDGCreate  DialogControllerArgs=DataTag29  SystemSampleTime=-1  Controller=PID  TimeDomain=Discrete-time  SampleTime=Ts  IntegratorMethod=Forward Euler  FilterMethod=Forward Euler  Form=Ideal  P=60  I=0.5  D=0  N=0  InitialConditionSource=internal  InitialConditionForIntegrator=0  InitialConditionForFilter=0  ExternalReset=none  ZeroCross=off  LimitOutput=off  UpperSaturationLimit=inf  LowerSaturationLimit=-inf  LinearizeAsGain=off  AntiWindupMode=none  Kb=1  TrackingMode=off  Kt=1  PParamMin=[]  PParamMax=[]  IParamMin=[]  IParamMax=[]  DParamMin=[]  DParamMax=[]  NParamMin=[]  NParamMax=[]  KbParamMin=[]  KbParamMax=[]  KtParamMin=[]  KtParamMax=[]  POutMin=[]  POutMax=[]  IOutMin=[]  IOutMax=[]  DOutMin=[]  DOutMax=[]  NOutMin=[]  NOutMax=[]  KbOutMin=[]  KbOutMax=[]  KtOutMin=[]  KtOutMax=[]  IntegratorOutMin=[]  IntegratorOutMax=[]  FilterOutMin=[]  FilterOutMax=[]  SumOutMin=[]  SumOutMax=[]  SumI1OutMin=[]  SumI1OutMax=[]  SumI2OutMin=[]  SumI2OutMax=[]  SumI3OutMin=[]  SumI3OutMax=[]  SumDOutMin=[]  SumDOutMax=[]  SaturationOutMin=[]  SaturationOutMax=[]  IntegratorContinuousStateAttributes=''  IntegratorStateMustResolveToSignalObject=off  IntegratorRTWStateStorageClass=Auto  FilterContinuousStateAttributes=''  FilterStateMustResolveToSignalObject=off  FilterRTWStateStorageClass=Auto
  Saturation : Saturate  UpperLimit=255  LowerLimit=0  OutDataType=fixdt(1, 16)  OutScaling=2^0
  Sum : Sum  Inputs=|+-  OutDataType=fixdt(1, 16)  OutScaling=2^0
  Sum1 : Sum  Inputs=|+-  OutDataType=fixdt(1, 16)  OutScaling=2^0
  Sum{9..14} (6 alike) : Sum  Inputs=+-  OutDataType=fixdt(1, 16)  OutScaling=2^0
  Sum2 : Sum  Inputs=|++  OutDataType=fixdt(1, 16)  OutScaling=2^0
  Sum3 : Sum  Inputs=|+--  OutDataType=fixdt(1, 16)  OutScaling=2^0
  Sum4 : Sum  Inputs=|+++  OutDataType=fixdt(1, 16)  OutScaling=2^0
  Sum5 : Sum  Inputs=+-+  OutDataType=fixdt(1, 16)  OutScaling=2^0
  Sum6 : Sum  Inputs=++-  OutDataType=fixdt(1, 16)  OutScaling=2^0
  Sum7 : Sum  Inputs=+++  OutDataType=fixdt(1, 16)  OutScaling=2^0
  Sum8 : Sum  Inputs=+--  OutDataType=fixdt(1, 16)  OutScaling=2^0
  Terminator : Terminator
  y_out : Outport  OutDataType=fixdt(1, 16)  OutScaling=2^0
  wires:
  Gain4/1 -> Hover Mode Enable/3(r_psiSet), Sum2/1
  Sum9/1 -> Gain4/1
  [phi_ctrl] -> Sum3/1
  Sum14/1 -> Gain9/1
  Gain9/1 -> Sum4/2
  [theta_ctrl] -> Sum4/1
  Sum13/1 -> Gain7/1
  Gain7/1 -> Sum3/2
  Gain3/1 -> Sum1/1, Hover Mode Enable/1(phiSet)
  Gain2/1 -> Sum/1, Hover Mode Enable/2(thetaSet)
  Sum11/1 -> Gain2/1
  Sum10/1 -> Gain3/1
  [r_theta] -> Sum14/1
  Constant5/1 -> Sum14/2
  [r_phi] -> Sum13/1
  Constant4/1 -> Sum13/2
  Constant2/1 -> Sum11/2
  [theta_set] -> Sum11/1
  Constant1/1 -> Sum10/2
  [phi_set] -> Sum10/1
  Constant/1 -> Sum9/2
  [rpsi_set] -> Sum9/1
  Saturation/1 -> y_out/1
  Mux/1 -> Saturation/1
  [m_psi] -> Sum8/3
  [m_phi] -> Sum8/2
  [m_psi] -> Sum7/3
  [m_theta] -> Sum7/2
  [m_psi] -> Sum6/3
  [m_phi] -> Sum6/2
  [m_psi] -> Sum5/3
  [m_theta] -> Sum5/2
  [thrust_set] -> Sum8/1, Sum7/1, Sum6/1, Sum5/1
  PID rTheta/1 -> [m_theta]
  PID rPhi/1 -> [m_phi]
  PID Theta/1 -> [theta_ctrl]
  PID Phi/1 -> [phi_ctrl]
  Sum6/1 -> Mux/2  "M2"
  Sum7/1 -> Mux/3  "M3"
  Sum8/1 -> Mux/4  "M4"
  Sum5/1 -> Mux/1  "M1"
  Sum4/1 -> PID rTheta/1  "e_r_theta"
  Sum3/1 -> PID rPhi/1  "e_r_phi"
  Sum2/1 -> PID rPsi/1  "e_r_psi"
  Sum1/1 -> PID Phi/1  "e_phi"
  [phi] -> Sum1/2
  Sum/1 -> PID Theta/1  "e_theta"
  [theta] -> Sum/2
  Gain1/1 -> [phi]
  Gain/1 -> [theta]
  Demux/9 -> [thrust_set]
  Demux/8 -> [rpsi_set]
  Demux/7 -> [theta_set]
  Demux/6 -> [phi_set]
  Demux/5 -> [r_psi]
  Demux/4 -> [r_theta]
  Demux/3 -> [r_phi]
  Demux/1 -> Gain/1
  Demux/2 -> Gain1/1
  u_in/1 -> Demux/1
  Demux/10 -> [vx_opt]
  Demux/11 -> [vy_opt]
  Demux/12 -> [rpsi_opt]
  [vy_opt] -> Control Hovering Mode/4(vy_opt)
  [vx_opt] -> Control Hovering Mode/1(vx_opt)
  [rpsi_opt] -> Control Hovering Mode/5(rpsi_opt)
  Control Hovering Mode/1(m_theta) -> Sum4/3
  Control Hovering Mode/2(m_phi) -> Sum3/3
  Constant7/1 -> Hover Mode Enable/4(set_val_th)
  Gain5/1 -> Sum2/2
  Sum12/1 -> Gain5/1
  Constant3/1 -> Sum12/2
  [r_psi] -> Sum12/1
  Constant6/1 -> Control Hovering Mode/2(theta_hm_set), Control Hovering Mode/3(phi_hm_set), Control Hovering Mode/6(rpsi_hm_set)
  PID rPsi/1 -> [m_psi]
  Hover Mode Enable/1(Control) -> Control Hovering Mode/Enable
  Control Hovering Mode/3(m_psi) -> Terminator/1

== system System_Design_Quadrocopter/Quadrocopter/Dynamics/Brushless_Motor1 ==
  note: Brushless Motor
  note: Gain of BLDC
  Set-Point_in : Inport  OutDataType=fixdt(1, 16)  OutScaling=2^0
  Data Type Conversion : DataTypeConversion  OutDataTypeMode=double  OutDataType=fixdt(1, 16)  OutScaling=2^0  OutDataTypeStr=double
  Gain6 : Gain  Gain=M_error  ParameterDataType=fixdt(1, 16)  ParameterScaling=2^0  OutDataType=fixdt(1, 16)  OutScaling=2^0
  Motor Delay : TransferFcn  Denominator=[0.001 1]  ContinuousStateAttributes='Motor_Delay'
  Saturation : Saturate  UpperLimit=255  LowerLimit=0  OutDataType=fixdt(1, 16)  OutScaling=2^0
  Set-point to Thrust : Lookup  InputValues=[0 40 175]  Table=[0 500 4500]./1000  LookUpMeth=Interpolation-Use End Values  OutDataType=fixdt(1, 16)  OutScaling=2^0
  Thrust to rpm : Lookup  InputValues=thrust  Table=speed  LookUpMeth=Interpolation-Use End Values  OutDataType=fixdt(1, 16)  OutScaling=2^0
  anv_prop_out : Outport  OutDataType=fixdt(1, 16)  OutScaling=2^0
  F_prop_out : Outport  Port=2  OutDataType=fixdt(1, 16)  OutScaling=2^0
  wires:
  Thrust to rpm/1 -> anv_prop_out/1
  Gain6/1 -> Thrust to rpm/1, F_prop_out/1
  Motor Delay/1 -> Gain6/1
  Data Type Conversion/1 -> Set-point to Thrust/1
  Set-Point_in/1 -> Saturation/1
  Saturation/1 -> Data Type Conversion/1
  Set-point to Thrust/1 -> Motor Delay/1

== system System_Design_Quadrocopter/Quadrocopter/Dynamics/Brushless_Motor3 ==
  note: Brushless Motor (new Continuous)
  note: Verrzögerung des Kraft
  note: Registerwert in Kraft umsetzten
  note: Kraft in Drehzahl umrechnen
  note: Gain of BLDC
  anv_prob : Inport  OutDataType=fixdt(1, 16)  OutScaling=2^0
  Data Type Conversion : DataTypeConversion  OutDataTypeMode=double  OutDataType=fixdt(1, 16)  OutScaling=2^0  OutDataTypeStr=double
  Gain6 : Gain  Gain=M_error  ParameterDataType=fixdt(1, 16)  ParameterScaling=2^0  OutDataType=fixdt(1, 16)  OutScaling=2^0
  Motor_Delay : TransferFcn  Denominator=[0.001 1]  ContinuousStateAttributes='Motor_Delay'
  Saturation : Saturate  UpperLimit=255  LowerLimit=0  OutDataType=fixdt(1, 16)  OutScaling=2^0
  setpoint_thrust_prop : Lookup  InputValues=[0 40 175]  Table=[0 500 4500]./1000  LookUpMeth=Interpolation-Use End Values  OutDataType=fixdt(1, 16)  OutScaling=2^0
  thrust_speed_prop : Lookup  InputValues=thrust  Table=speed  LookUpMeth=Interpolation-Use End Values  OutDataType=fixdt(1, 16)  OutScaling=2^0
  anv_prop1 : Outport  OutDataType=fixdt(1, 16)  OutScaling=2^0
  F_prop1 : Outport  Port=2  OutDataType=fixdt(1, 16)  OutScaling=2^0
  wires:
  thrust_speed_prop/1 -> anv_prop1/1
  Gain6/1 -> thrust_speed_prop/1, F_prop1/1
  Motor_Delay/1 -> Gain6/1
  Data Type Conversion/1 -> setpoint_thrust_prop/1
  anv_prob/1 -> Saturation/1
  Saturation/1 -> Data Type Conversion/1
  setpoint_thrust_prop/1 -> Motor_Delay/1

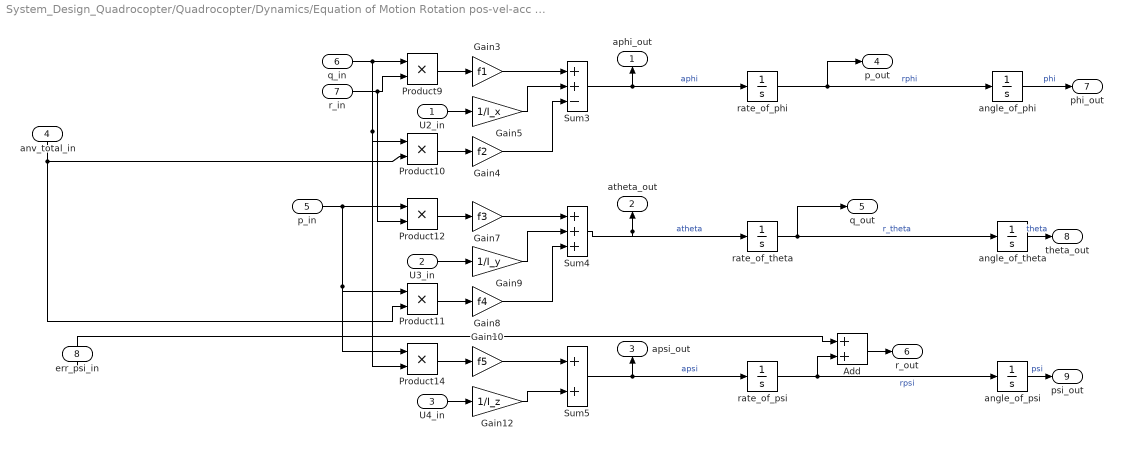
== system System_Design_Quadrocopter/Quadrocopter/Dynamics/Equation of Motion Rotation pos-vel-acc B-frame ==
  U2_in : Inport
  U3_in : Inport  Port=2
  U4_in : Inport  Port=3
  anv_total_in : Inport  Port=4
  p_in : Inport  Port=5
  q_in : Inport  Port=6
  r_in : Inport  Port=7
  err_psi_in : Inport  Port=8
  Add : Sum  OutDataType=fixdt(1, 16)  OutScaling=2^-10
  Gain10 : Gain  Gain=f5
  Gain12 : Gain  Gain=1/I_z
  Gain3 : Gain  Gain=f1
  Gain4 : Gain  Gain=f2
  Gain5 : Gain  Gain=1/I_x
  Gain7 : Gain  Gain=f3
  Gain8 : Gain  Gain=f4
  Gain9 : Gain  Gain=1/I_y
  Product{9..12,14} (5 alike) : Product  RndMeth=Zero
  Sum3 : Sum  Inputs=++-
  Sum4 : Sum  Inputs=+++
  Sum5 : Sum
  angle_of_phi : Integrator  InitialCondition=phi0
  angle_of_psi : Integrator
  angle_of_theta : Integrator  InitialCondition=theta0
  rate_of_phi : Integrator  InitialCondition=r_phi0
  rate_of_psi : Integrator  InitialCondition=r_psi0
  rate_of_theta : Integrator  InitialCondition=r_theta0
  aphi_out : Outport
  atheta_out : Outport  Port=2
  apsi_out : Outport  Port=3
  p_out : Outport  Port=4
  q_out : Outport  Port=5
  r_out : Outport  Port=6
  phi_out : Outport  Port=7
  theta_out : Outport  Port=8
  psi_out : Outport  Port=9
  wires:
  p_in/1 -> Product14/1, Product11/1, Product12/1
  r_in/1 -> Product12/2, Product9/2
  q_in/1 -> Product14/2, Product10/1, Product9/1
  rate_of_psi/1 -> angle_of_psi/1, Add/2  "rpsi"
  rate_of_theta/1 -> angle_of_theta/1, q_out/1  "r_theta"
  rate_of_phi/1 -> angle_of_phi/1, p_out/1  "rphi"
  anv_total_in/1 -> Product10/2, Product11/2
  Product9/1 -> Gain3/1
  Gain3/1 -> Sum3/1
  Product10/1 -> Gain4/1
  Gain5/1 -> Sum3/2
  Gain4/1 -> Sum3/3
  Sum3/1 -> rate_of_phi/1, aphi_out/1  "aphi"
  Product12/1 -> Gain7/1
  Gain7/1 -> Sum4/1
  Product11/1 -> Gain8/1
  Gain9/1 -> Sum4/2
  Gain8/1 -> Sum4/3
  Sum4/1 -> rate_of_theta/1, atheta_out/1  "atheta"
  Product14/1 -> Gain10/1
  Gain10/1 -> Sum5/1
  Gain12/1 -> Sum5/2
  Sum5/1 -> rate_of_psi/1, apsi_out/1  "apsi"
  angle_of_phi/1 -> phi_out/1  "phi"
  U2_in/1 -> Gain5/1
  angle_of_theta/1 -> theta_out/1  "theta"
  U3_in/1 -> Gain9/1
  angle_of_psi/1 -> psi_out/1  "psi"
  U4_in/1 -> Gain12/1
  Add/1 -> r_out/1
  err_psi_in/1 -> Add/1

== system System_Design_Quadrocopter/Quadrocopter/Dynamics/Equation of Motion Translation pos-vel-acc B-Frame ==
  vxe : Inport
  vye : Inport  Port=2
  vze : Inport  Port=3
  phie : Inport  Port=4
  thetae : Inport  Port=5
  psie : Inport  Port=6
  Equation of Motion Translation vel B-Frame : Subsystem
  u : Outport
  v : Outport  Port=2
  w : Outport  Port=3
  wires:
  Equation of Motion Translation vel B-Frame/1(u) -> u/1
  Equation of Motion Translation vel B-Frame/3(w) -> w/1
  Equation of Motion Translation vel B-Frame/2(v) -> v/1
  vxe/1 -> Equation of Motion Translation vel B-Frame/1(vxe)
  vye/1 -> Equation of Motion Translation vel B-Frame/2(vye)
  vze/1 -> Equation of Motion Translation vel B-Frame/3(vze)
  phie/1 -> Equation of Motion Translation vel B-Frame/4(phi)
  thetae/1 -> Equation of Motion Translation vel B-Frame/5(theta)
  psie/1 -> Equation of Motion Translation vel B-Frame/6(psi)

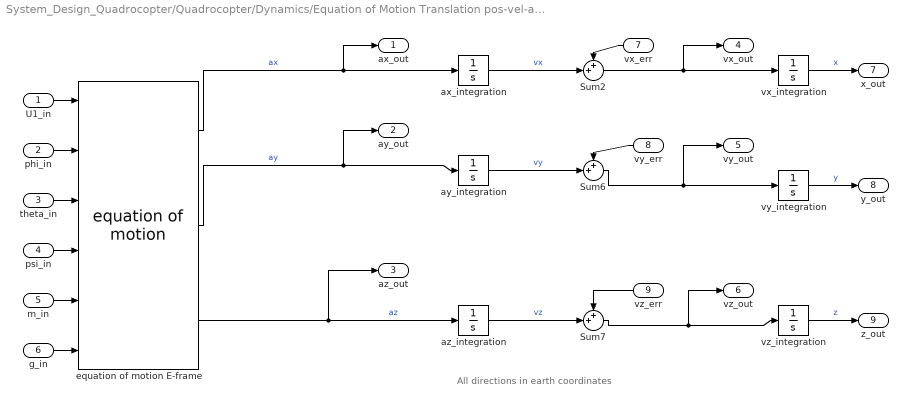
== system System_Design_Quadrocopter/Quadrocopter/Dynamics/Equation of Motion Translation pos-vel-acc E-frame ==
  note: All directions in earth coordinates
  U1_in : Inport
  phi_in : Inport  Port=2
  theta_in : Inport  Port=3
  psi_in : Inport  Port=4
  m_in : Inport  Port=5
  g_in : Inport  Port=6
  vx_err : Inport  Port=7
  vy_err : Inport  Port=8
  vz_err : Inport  Port=9
  Sum2 : Sum  Inputs=++|
  Sum6 : Sum  Inputs=++|
  Sum7 : Sum  Inputs=++|
  ax_integration : Integrator
  ay_integration : Integrator
  az_integration : Integrator
  equation of motion E-frame : Copter_Library/equation of motion  SystemSampleTime=-1
  vx_integration : Integrator
  vy_integration : Integrator
  vz_integration : Integrator
  ax_out : Outport
  ay_out : Outport  Port=2
  az_out : Outport  Port=3
  vx_out : Outport  Port=4
  vy_out : Outport  Port=5
  vz_out : Outport  Port=6
  x_out : Outport  Port=7
  y_out : Outport  Port=8
  z_out : Outport  Port=9
  wires:
  equation of motion E-frame/2 -> ay_integration/1, ay_out/1  "ay"
  equation of motion E-frame/1 -> ax_integration/1, ax_out/1  "ax"
  Sum2/1 -> vx_integration/1, vx_out/1
  ay_integration/1 -> Sum6/2  "vy"
  Sum6/1 -> vy_integration/1, vy_out/1
  az_integration/1 -> Sum7/2  "vz"
  equation of motion E-frame/3 -> az_integration/1, az_out/1  "az"
  Sum7/1 -> vz_integration/1, vz_out/1
  ax_integration/1 -> Sum2/2  "vx"
  U1_in/1 -> equation of motion E-frame/1
  vx_err/1 -> Sum2/1
  vx_integration/1 -> x_out/1  "x"
  phi_in/1 -> equation of motion E-frame/2
  theta_in/1 -> equation of motion E-frame/3
  vy_err/1 -> Sum6/1
  psi_in/1 -> equation of motion E-frame/4
  vy_integration/1 -> y_out/1  "y"
  m_in/1 -> equation of motion E-frame/5
  vz_err/1 -> Sum7/1
  g_in/1 -> equation of motion E-frame/6
  vz_integration/1 -> z_out/1  "z"

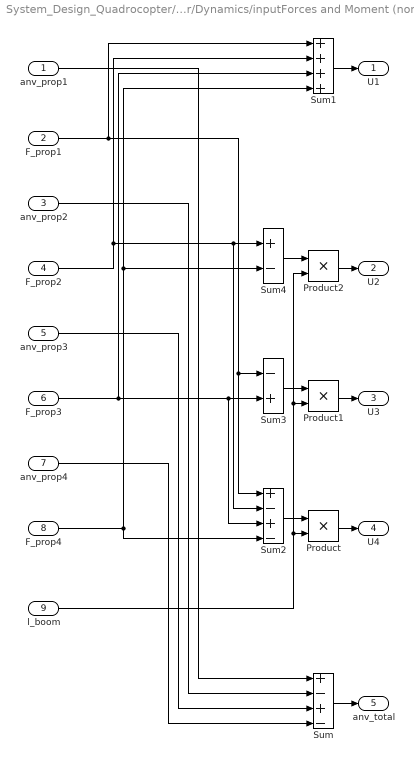
== system System_Design_Quadrocopter/Quadrocopter/Dynamics/inputForces and Moment (non Emb) ==
  anv_prop1 : Inport  OutDataType=fixdt(1, 16)  OutScaling=2^0
  F_prop1 : Inport  Port=2  OutDataType=fixdt(1, 16)  OutScaling=2^0
  anv_prop2 : Inport  Port=3  OutDataType=fixdt(1, 16)  OutScaling=2^0
  F_prop2 : Inport  Port=4  OutDataType=fixdt(1, 16)  OutScaling=2^0
  anv_prop3 : Inport  Port=5  OutDataType=fixdt(1, 16)  OutScaling=2^0
  F_prop3 : Inport  Port=6  OutDataType=fixdt(1, 16)  OutScaling=2^0
  anv_prop4 : Inport  Port=7  OutDataType=fixdt(1, 16)  OutScaling=2^0
  F_prop4 : Inport  Port=8  OutDataType=fixdt(1, 16)  OutScaling=2^0
  l_boom : Inport  Port=9  OutDataType=fixdt(1, 16)  OutScaling=2^0
  Product : Product  OutDataType=fixdt(1, 16)  OutScaling=2^0  RndMeth=Zero
  Product1 : Product  OutDataType=fixdt(1, 16)  OutScaling=2^0  RndMeth=Zero
  Product2 : Product  OutDataType=fixdt(1, 16)  OutScaling=2^0  RndMeth=Zero
  Sum : Sum  Inputs=+-+-  OutDataType=fixdt(1, 16)  OutScaling=2^0
  Sum1 : Sum  Inputs=++++  OutDataType=fixdt(1, 16)  OutScaling=2^0
  Sum2 : Sum  Inputs=+-+-  OutDataType=fixdt(1, 16)  OutScaling=2^0
  Sum3 : Sum  Inputs=-+  OutDataType=fixdt(1, 16)  OutScaling=2^0
  Sum4 : Sum  Inputs=+-  OutDataType=fixdt(1, 16)  OutScaling=2^0
  U1 : Outport  OutDataType=fixdt(1, 16)  OutScaling=2^0
  U2 : Outport  Port=2  OutDataType=fixdt(1, 16)  OutScaling=2^0
  U3 : Outport  Port=3  OutDataType=fixdt(1, 16)  OutScaling=2^0
  U4 : Outport  Port=4  OutDataType=fixdt(1, 16)  OutScaling=2^0
  anv_total : Outport  Port=5  OutDataType=fixdt(1, 16)  OutScaling=2^0
  wires:
  Product/1 -> U4/1
  Product1/1 -> U3/1
  Product2/1 -> U2/1
  Sum2/1 -> Product/1
  Sum3/1 -> Product1/1
  Sum4/1 -> Product2/1
  l_boom/1 -> Product2/2, Product1/2, Product/2
  F_prop4/1 -> Sum2/4, Sum4/2, Sum1/4
  F_prop3/1 -> Sum2/3, Sum3/2, Sum1/3
  F_prop2/1 -> Sum2/2, Sum4/1, Sum1/2
  F_prop1/1 -> Sum2/1, Sum3/1, Sum1/1
  Sum1/1 -> U1/1
  anv_prop1/1 -> Sum/1
  anv_prop2/1 -> Sum/2
  anv_prop3/1 -> Sum/3
  anv_prop4/1 -> Sum/4
  Sum/1 -> anv_total/1

== system System_Design_Quadrocopter/Quadrocopter/Remote Control/Const_Stimuli ==
  note: phi(roll)
      | theta(pitch)
      | rpsi(yaw rate)
      | T(thrust)
  phi : Inport  OutDataType=fixdt(1, 16)  OutScaling=2^0
  theta : Inport  Port=2  OutDataType=fixdt(1, 16)  OutScaling=2^0
  rpsi : Inport  Port=3  OutDataType=fixdt(1, 16)  OutScaling=2^0
  Add : Sum  OutDataType=fixdt(1, 16)  OutScaling=2^-10
  Add1 : Sum  OutDataType=fixdt(1, 16)  OutScaling=2^-10
  Add2 : Sum  OutDataType=fixdt(1, 16)  OutScaling=2^-10
  Constant{,1..3} (4 alike) : Constant  Value=128  OutDataType=fixdt(1, 16)  OutScaling=2^0
  Gain : Gain  ParameterDataType=fixdt(1, 16)  ParameterScaling=2^0  OutDataType=fixdt(1, 16)  OutScaling=2^0
  Mux1 : Mux
  Out : Outport  OutDataType=fixdt(1, 16)  OutScaling=2^0
  wires:
  Mux1/1 -> Out/1
  Constant/1 -> Gain/1
  Gain/1 -> Mux1/4  "thrust"
  Constant3/1 -> Add/2
  phi/1 -> Add/1
  Constant1/1 -> Add1/2
  theta/1 -> Add1/1
  Constant2/1 -> Add2/2  "rpsi_set"
  rpsi/1 -> Add2/1
  Add/1 -> Mux1/1
  Add1/1 -> Mux1/2
  Add2/1 -> Mux1/3
